simulink library "SimulinkMATPOWERbase"  (R2020b)
settings: Solver=ode45  StartTime=0.0  StopTime=10.0  RelTol=1e-3
settings Model: Creator=hauswirth  LastModifiedBy=lukas
settings DataIOCC: SaveFormat=StructureWithTime  ReturnWorkspaceOutputs=off
settings OptimizationCC: LifeSpan=inf
settings DebuggingCC: SFExecutionAtInitializationDiag=none  ArithmeticOperatorsInVariantConditions=warning
settings HardwareCC: ProdBitPerSizeT=32  ProdBitPerPtrDiffT=32  ProdWordSize=32  ProdHWDeviceType=Specified
settings SFSimCC: CustomCodeUndefinedFunction=UseInterfaceOnly
settings CodeAppCC: StateflowObjectComments=on

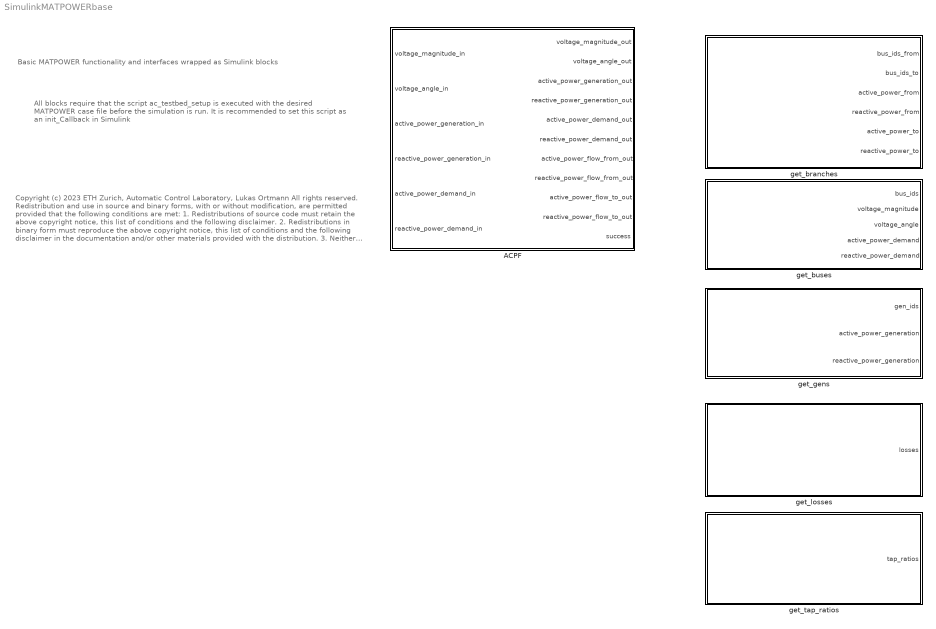
== system SimulinkMATPOWERbase ==
  note: Copyright (c) 2023 ETH Zurich, Automatic Control Laboratory, Lukas Ortmann
      | All rights reserved.
      |
      | Redistribution and use in source and binary forms, with or without
      | modification, are permitted provided that the following conditions are
      | met:
      |
      | 1. Redistributions of source code must retain the above copyright
      | notice, this list of conditions and the following disclaimer.
      |
      | 2. Redistributions in binary form must reproduce the above copyright
      | notice, this list of conditions and the following disclaimer in the
      | documentation and/or other materials provided with the distribution.
      |
      | 3. Neither the name of the copyright holder nor the names of its
      | contributors may be used to endorse or promote products derived from
      | this software without specific prior written permission.
      |
      | THIS SOFTWARE IS PROVIDED BY THE COPYRIGHT HOLDERS AND CONTRIBUTORS "AS
      | IS" AND ANY EXPRESS OR IMPLIED WARRANTIES, INCLUDING, BUT NOT LIMITED
      | TO, THE IMPLIED WARRANTIES OF MERCHANTABILITY AND FITNESS FOR A
      | PARTICULAR PURPOSE ARE DISCLAIMED. IN NO EVENT SHALL THE COPYRIGHT
      | HOLDER OR CONTRIBUTORS BE LIABLE FOR ANY DIRECT, INDIRECT, INCIDENTAL,
      | SPECIAL, EXEMPLARY, OR CONSEQUENTIAL DAMAGES (INCLUDING, BUT NOT LIMITED
      | TO, PROCUREMENT OF SUBSTITUTE GOODS OR SERVICES; LOSS OF USE, DATA, OR
      | PROFITS; OR BUSINESS INTERRUPTION) HOWEVER CAUSED AND ON ANY THEORY OF
      | LIABILITY, WHETHER IN CONTRACT, STRICT LIABILITY, OR TORT (INCLUDING
      | NEGLIGENCE OR OTHERWISE) ARISING IN ANY WAY OUT OF THE USE OF THIS
      | SOFTWARE, EVEN IF ADVISED OF THE POSSIBILITY OF SUCH DAMAGE.
  note: All blocks require that the script ac_testbed_setup is
      | executed with the desired MATPOWER case file before the
      | simulation is run. It is recommended to set this script
      | as an init_Callback in Simulink
  note: Basic MATPOWER functionality and
      | interfaces wrapped as Simulink blocks
  ACPF : MATLAB Function  TreatAsAtomicUnit=on
  get_branches : MATLAB Function  TreatAsAtomicUnit=on  SystemSampleTime=1
  get_buses : MATLAB Function  TreatAsAtomicUnit=on  SystemSampleTime=1
  get_gens : MATLAB Function  TreatAsAtomicUnit=on  SystemSampleTime=1
  get_losses : MATLAB Function  TreatAsAtomicUnit=on  SystemSampleTime=1
  get_tap_ratios : MATLAB Function  TreatAsAtomicUnit=on  SystemSampleTime=1

== matlab function SimulinkMATPOWERbase/get_gens ==
  data: gen_ids output; active_power_generation output; reactive_power_generation output; zeros_num_gens parameter
function [gen_ids, active_power_generation, reactive_power_generation] ...
    = get_gens_wrapper(zeros_num_gens)
%% Wrapper function to access get_generators function

% Roger Germann, Kerry Jansen, Denis Mikhaylov 02-05.2020
    
    %% Allocate memory to return values  
    % Dynamic memory allocation is not possible with extrinsic functions.
    % Therefore the dimensions need to be set by hand. The output size is
    % predefined in ac_testbed_setup.m
    gen_ids  = zeros_num_gens;
    active_power_generation = zeros_num_gens;
    reactive_power_generation = zeros_num_gens;

    
    %% Define get_blocaux_generators as extrinsic 
    % - to avoid code generation
    % - to allow the use of evalin and assignin
    % - in order to use sparse matrices and avoid passing these to simulink
    coder.extrinsic('get_generators');
    
    %% Call extrinsic function and return results. 
    [gen_ids, active_power_generation, reactive_power_generation]=get_generators();
end

== matlab function SimulinkMATPOWERbase/get_tap_ratios ==
  data: tap_ratios output; zeros_num_tap_ratios parameter
function tap_ratios = get_tap_ratios_wrapper(zeros_num_tap_ratios)
%% Wrapper function to access get_tap_ratios function

% Lukas Ortmann 23.11.2020

    %% Allocate memory to return values  
    % Dynamic memory allocation is not possible with extrinsic functions.
    % Therefore the dimensions need to be set by hand. The output size is
    % predefined in ac_testbed_setup.m
    tap_ratios = zeros_num_tap_ratios;
    
    %% Define get_tap_ratios as extrinsic 
    % - to avoid code generation
    coder.extrinsic('get_tap_ratios');
    
    %% Call extrinsic function and return results. 
    tap_ratios = get_tap_ratios();
end

== matlab function SimulinkMATPOWERbase/ACPF ==
  data: voltage_magnitude_out output; voltage_angle_out output; active_power_generation_out output; reactive_power_generation_out output; active_power_demand_out output; reactive_power_demand_out output; active_power_flow_from_out output size=number_branches; reactive_power_flow_from_out output size=number_branches; active_power_flow_to_out output size=number_branches; reactive_power_flow_to_out output size=number_branches; voltage_magnitude_in input; voltage_angle_in input; active_power_generation_in input; reactive_power_generation_in input; success output size=1; active_power_demand_in input; reactive_power_demand_in input; zeros_num_branches parameter
function [voltage_magnitude_out, voltage_angle_out, active_power_generation_out, reactive_power_generation_out, active_power_demand_out, reactive_power_demand_out, active_power_flow_from_out, reactive_power_flow_from_out, active_power_flow_to_out, reactive_power_flow_to_out, success] ...
    = ACPF(voltage_magnitude_in, voltage_angle_in, active_power_generation_in, reactive_power_generation_in, active_power_demand_in, reactive_power_demand_in, zeros_num_branches)
%% Wrapper function for extrinsic_ACPF which in turn implements runpf from
%% MATPOWER

% Roger Germann, Kerry Jansen, Denis Mikhaylov 02-05.2020

    %% Allocate memory to return values  
    % Dynamic memory allocation is not possible with extrinsic functions. 
    voltage_magnitude_out = zeros(size(voltage_magnitude_in));
    voltage_angle_out = zeros(size(voltage_angle_in));
    active_power_generation_out = zeros(size(active_power_generation_in));
    reactive_power_generation_out = zeros(size(reactive_power_generation_in));
    active_power_demand_out = zeros(size(active_power_demand_in));
    reactive_power_demand_out = zeros(size(reactive_power_demand_in));
    active_power_flow_from_out = zeros_num_branches;
    reactive_power_flow_from_out = zeros_num_branches;
    active_power_flow_to_out = zeros_num_branches;
    reactive_power_flow_to_out = zeros_num_branches;
    success = 0;
    
    %% Define extrinsic_ACPF as extrinsic 
    % - to avoid code generation
    % - to allow the use of evalin and assignin
    % - in order to use sparse matrices and avoid passing these to simulink
    coder.extrinsic('extrinsic_ACPF');
    
    %% Call extrinsic function and return results. 
    [voltage_magnitude_out, voltage_angle_out, active_power_generation_out, reactive_power_generation_out, active_power_demand_out,reactive_power_demand_out, active_power_flow_from_out, reactive_power_flow_from_out, active_power_flow_to_out, reactive_power_flow_to_out, success]=extrinsic_ACPF(voltage_magnitude_in, voltage_angle_in, active_power_generation_in, reactive_power_generation_in, active_power_demand_in, reactive_power_demand_in);
    
    %% check whether or not the power flow was successfully solved
    if success ~= 1
       error('Power Flow not successfully solved'); 
    end
end

== matlab function SimulinkMATPOWERbase/get_buses ==
  data: bus_ids output; voltage_magnitude output; voltage_angle output; active_power_demand output; reactive_power_demand output; zeros_num_buses parameter
function [bus_ids, voltage_magnitude, voltage_angle, active_power_demand, reactive_power_demand] ...
    = get_buses_wrapper(zeros_num_buses)
%% Wrapper function to access get_buses function

% Roger Germann, Kerry Jansen, Denis Mikhaylov 02-05.2020
    
        %% Allocate memory to return values  
    % Dynamic memory allocation is not possible with extrinsic functions.
    % Therefore the dimensions need to be set by hand. The output size is
    % predefined in ac_testbed_setup.m
    bus_ids  = zeros_num_buses;
    voltage_magnitude = zeros_num_buses;
    voltage_angle = zeros_num_buses;
    active_power_demand = zeros_num_buses;
    reactive_power_demand = zeros_num_buses;

    
    %% Define get_blocaux_buses as extrinsic 
    % - to avoid code generation
    % - to allow the use of evalin and assignin
    % - in order to use sparse matrices and avoid passing these to simulink
    coder.extrinsic('get_buses');
    
    %% Call extrinsic function and return results. 
    [bus_ids, voltage_magnitude, voltage_angle, active_power_demand, reactive_power_demand]=get_buses();
end

== matlab function SimulinkMATPOWERbase/get_losses ==
  data: losses output size=1
function losses = get_losses_wrapper()
%% Wrapper function get the losses

% Lukas Ortmann 23-07.2021
    
    %% Allocate memory to return values  
    % Dynamic memory allocation is not possible with extrinsic functions.
    % Therefore the dimensions need to be set by hand by assigning zero
    losses = 0;
    %% Define get_losses_all_blocaux as extrinsic 
    % - to avoid code generation
    % - to allow the use of evalin and assignin
    % - in order to use sparse matrices and avoid passing these to simulink
    coder.extrinsic('get_losses_from_matpower');
    
    %% Call extrinsic function and return results. 
    losses = get_losses_from_matpower();
end

== matlab function SimulinkMATPOWERbase/get_branches ==
  data: bus_ids_from output; bus_ids_to output; active_power_from output; reactive_power_from output; active_power_to output; reactive_power_to output; zeros_num_branches parameter
 function [bus_ids_from, bus_ids_to, active_power_from, reactive_power_from, active_power_to, reactive_power_to] ...
    = get_branches_wrapper(zeros_num_branches)
%% Wrapper function to access get_branches function

% Roger Germann, Kerry Jansen, Denis Mikhaylov 02-05.2020

    %% Allocate memory to return values  
    % Dynamic memory allocation is not possible with extrinsic functions.
    % Therefore the dimensions need to be set by hand. The output size is
    % predefined in ac_testbed_setup.m
    bus_ids_from = zeros_num_branches;
    bus_ids_to = zeros_num_branches;
    active_power_from = zeros_num_branches;
    reactive_power_from = zeros_num_branches;
    active_power_to = zeros_num_branches;
    reactive_power_to = zeros_num_branches;
    
    %% Define get_blocaux_branches as extrinsic 
    % - to avoid code generation
    % - to allow the use of evalin and assignin
    % - in order to use sparse matrices and avoid passing these to simulink
    coder.extrinsic('get_branches');
    
    %% Call extrinsic function and return results. 
    [bus_ids_from, bus_ids_to, active_power_from, reactive_power_from, active_power_to, reactive_power_to] = get_branches();
end
